simulink model "diff_eq"  (R2017b)
settings: Solver=VariableStepAuto  StartTime=0.0  StopTime=10.0  RelTol=1e-3
settings Model: Creator=nadav  LastModifiedBy=nadav

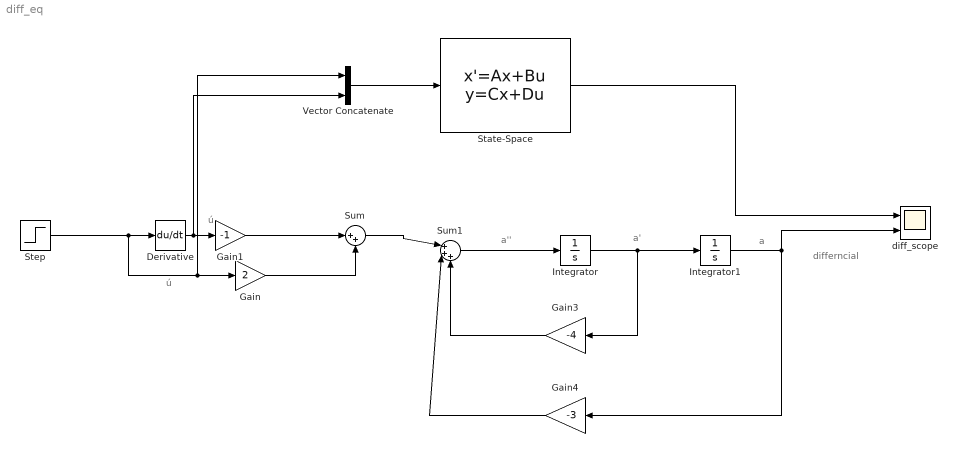
== system diff_eq ==
  note: differncial
  note: ú
  note: ú
  note: a
  note: a'
  note: a''
  Derivative : Derivative
  Gain : Gain  Gain=2
  Gain1 : Gain  Gain=-1
  Gain3 : Gain  Gain=-4
  Gain4 : Gain  Gain=-3
  Integrator : Integrator  InitialCondition=1
  Integrator1 : Integrator
  State-Space : StateSpace  A=[0 1; -3 -4]  B=[0 0; 2 -1]  C=[1 0]  D=[0 0]  InitialCondition=[0.5 0]
  Step : Step  Time=0  SampleTime=0
  Sum : Sum  Inputs=|++
  Sum1 : Sum  Inputs=|+++
  Vector Concatenate : Concatenate
  diff_scope : Scope  NumInputPorts=2
  wires:
  Step/1 -> Vector Concatenate/1, Gain/1, Derivative/1
  Gain/1 -> Sum/2
  Sum1/1 -> Integrator/1
  Integrator/1 -> Gain3/1, Integrator1/1
  Integrator1/1 -> Gain4/1, diff_scope/2
  Gain3/1 -> Sum1/3
  Gain4/1 -> Sum1/2
  Sum/1 -> Sum1/1
  Vector Concatenate/1 -> State-Space/1
  Gain1/1 -> Sum/1
  Derivative/1 -> Vector Concatenate/2, Gain1/1
  State-Space/1 -> diff_scope/1
